simulink model "Cessna_6DOF_trim"  (Simulink 8.3)
settings: Solver=ode45  StartTime=0.0  StopTime=1000  RelTol=1e-5
values from neighbouring files (symbols this model uses):
  I_xx = 1285.31    [Initial_Cessna.m]
  I_yy = 1824.93    [Initial_Cessna.m]
  I_zz = 2666.893    [Initial_Cessna.m]
  p = 0    [Initial_Cessna.m]
  phi = 0    [Initial_Cessna.m]
  psi = 0    [Initial_Cessna.m]
  q = 0    [Initial_Cessna.m]
  r = 0    [Initial_Cessna.m]
  theta = alpha    [Initial_Cessna.m]
  v = V_trim*sin(beta)    [Initial_Cessna.m]
  w = V_trim*sin(alpha)*cos(beta)    [Initial_Cessna.m]
  x = 0    [Initial_Cessna.m]
  y = 0    [Initial_Cessna.m]
  z = 0    [Initial_Cessna.m]
libraries: aerolibobsolete x1, aerolibasang x1
settings Model: Creator=Pranav  LastModifiedBy=Pranav
settings OptimizationCC: ExpressionDepthLimit=2147483647
settings DebuggingCC: FcnCallInpInsideContextMsg=UseLocalSettings

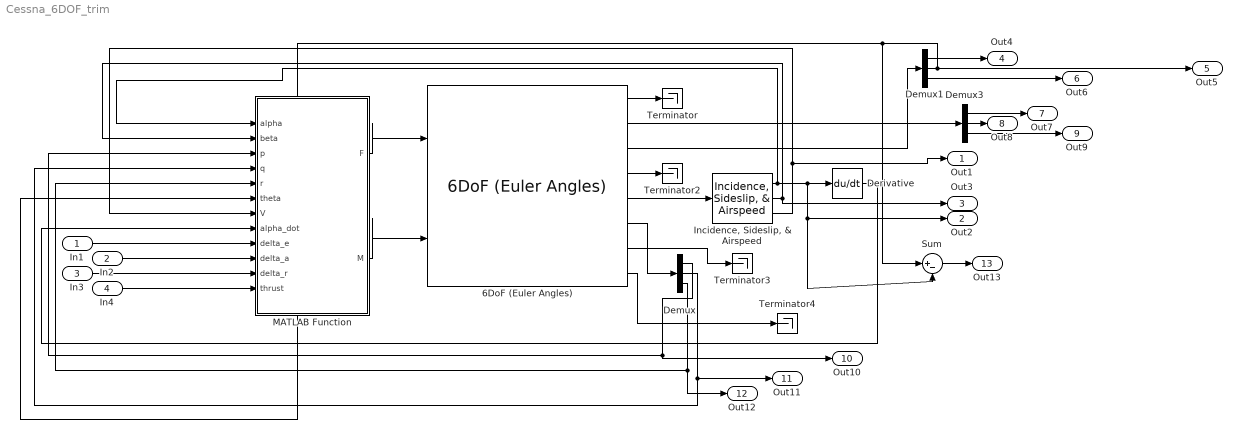
== system Cessna_6DOF_trim ==
  In1 : Inport
  In2 : Inport  Port=2
  In3 : Inport  Port=3
  In4 : Inport  Port=4
  6DoF (Euler Angles) : aerolibobsolete/6DoF (Euler Angles)  units=Metric (MKS)  mtype=Fixed  rep=Euler Angles  xme_0=[x y z]  Vm_0=[u v w]  eul_0=[phi theta psi]  pm_0=[p q r]  mass_0=m  mass_e=0.5  mass_f=2.0  inertia=diag([I_xx I_yy I_zz])  inertia_e=eye(3)  inertia_f=2*eye(3)  k_quat=1.0
  Demux : Demux  Outputs=3
  Demux1 : Demux  Outputs=3
  Demux3 : Demux  Outputs=3
  Derivative : Derivative
  "Incidence, Sideslip, & Airspeed" : aerolibasang/Incidence, Sideslip, & Airspeed
  MATLAB Function : MATLAB Function  TreatAsAtomicUnit=on
  Sum : Sum  Inputs=|+-
  Terminator{,2..4} (4 alike) : Terminator
  Out1 : Outport
  Out2 : Outport  Port=2
  Out3 : Outport  Port=3
  Out4 : Outport  Port=4
  Out5 : Outport  Port=5
  Out6 : Outport  Port=6
  Out7 : Outport  Port=7
  Out8 : Outport  Port=8
  Out9 : Outport  Port=9
  Out10 : Outport  Port=10
  Out11 : Outport  Port=11
  Out12 : Outport  Port=12
  Out13 : Outport  Port=13
  wires:
  6DoF (Euler Angles)/5 -> "Incidence, Sideslip, & Airspeed"/1
  6DoF (Euler Angles)/6 -> Demux/1
  MATLAB Function/1(F) -> 6DoF (Euler Angles)/1
  "Incidence, Sideslip, & Airspeed"/1 -> MATLAB Function/1(alpha), Derivative/1, Out2/1, Sum/2
  "Incidence, Sideslip, & Airspeed"/2 -> MATLAB Function/2(beta), Out3/1
  Demux/1 -> MATLAB Function/3(p), Out10/1
  Demux/2 -> MATLAB Function/4(q), Out11/1
  Demux/3 -> MATLAB Function/5(r), Out12/1
  "Incidence, Sideslip, & Airspeed"/3 -> MATLAB Function/7(V), Out1/1
  6DoF (Euler Angles)/1 -> Terminator/1
  6DoF (Euler Angles)/2 -> Demux3/1
  6DoF (Euler Angles)/4 -> Terminator2/1
  6DoF (Euler Angles)/7 -> Terminator3/1
  6DoF (Euler Angles)/8 -> Terminator4/1
  6DoF (Euler Angles)/3 -> Demux1/1
  Demux1/2 -> MATLAB Function/6(theta), Sum/1, Out5/1
  Demux1/1 -> Out4/1
  Demux1/3 -> Out6/1
  Demux3/1 -> Out7/1
  Demux3/2 -> Out8/1
  Demux3/3 -> Out9/1
  MATLAB Function/2(M) -> 6DoF (Euler Angles)/2
  Derivative/1 -> MATLAB Function/8(alpha_dot)
  Sum/1 -> Out13/1
  In1/1 -> MATLAB Function/9(delta_e)
  In2/1 -> MATLAB Function/10(delta_a)
  In3/1 -> MATLAB Function/11(delta_r)
  In4/1 -> MATLAB Function/12(thrust)

== matlab function MATLAB Function ==
  data: alpha input double; F output double; beta input double; p input double; q input double; r input double; theta input double; V input double; M output double; alpha_dot input double; delta_e input double; delta_a input double; delta_r input double; thrust input double
function [F, M] = Force_Cessna(alpha, beta, p, q, r, theta, V, alpha_dot, delta_e, delta_a, delta_r, thrust)

g = 9.8;
rho = 1.225;

m = 1043.26;
C_bar = 1.493;
b = 10.911;
S_ref = 16.1651;

C_L_0 = 0.25;
C_L_alpha = 4.47;
C_L_q = 1.7;
C_L_delta_e = 0.3476;

% Ignore all other C_D derivatives excluding C_D_0
% Use C_D = C_D_0 + k*C_L^2

C_D_0 = 0.036;
k = 0.3;

C_Y_beta = -0.31;
C_Y_p = -0.037;
C_Y_r = 0.21;
C_Y_delta_a = 0;

C_l_beta = -0.089;
C_l_p = -0.47;
C_l_r = 0.096;
C_l_delta_a = -0.09;
C_l_delta_r = 0.0147;

C_M_0 = -0.02;
C_M_alpha = -1.8;
C_M_alpha_dot = -12.4;
C_M_delta_e = -1.28;

C_N_beta = 0.065;
C_N_p = -0.03;
C_N_r = -0.99;
C_N_delta_a = -0.0053;
C_N_delta_r = -0.0657;

C_L = C_L_0 + C_L_alpha*alpha + C_L_q*(q*C_bar/(2*V)) + C_L_delta_e*delta_e;
C_D = C_D_0 + k*C_L^2;
C_Y = C_Y_beta*beta + C_Y_p*(p*b/(2*V)) + C_Y_r*(r*b/(2*V)) + C_Y_delta_a*delta_a;

C_l = C_l_beta*beta + C_l_p*(p*b/(2*V)) + C_l_r*(r*b/(2*V)) + C_l_delta_a*delta_a + C_l_delta_r*delta_r;
C_M = C_M_0 + C_M_alpha*alpha + C_M_alpha_dot*(alpha_dot*C_bar/(2*V)) + C_M_delta_e*delta_e;
C_N = C_N_beta*beta + C_N_p*(p*b/(2*V)) + C_N_r*(r*b/(2*V)) + C_N_delta_a*delta_a + C_N_delta_r*delta_r;

C_X = -C_D*cos(alpha) + C_L*sin(alpha);
C_Z = -C_D*sin(alpha) - C_L*cos(alpha);

F = zeros(3,1);
M = zeros(3,1);

q_bar = 0.5*rho*V*V;

F(1,1) = q_bar*S_ref*C_X - m*g*sin(theta) + thrust;
F(2,1) = q_bar*S_ref*C_Y;
F(3,1) = q_bar*S_ref*C_Z + m*g*cos(theta);

M(1,1) = q_bar*b*S_ref*C_l;
M(2,1) = q_bar*C_bar*S_ref*C_M;
M(3,1) = q_bar*b*S_ref*C_N;
